simulink model "sampleModel1947"  (R2023a)
settings: Solver=VariableStepAuto  StartTime=0.0  StopTime=10.0  RelTol=1e-3
libraries: hdlsllib x7
settings Model: Creator=user1  LastModifiedBy=user1

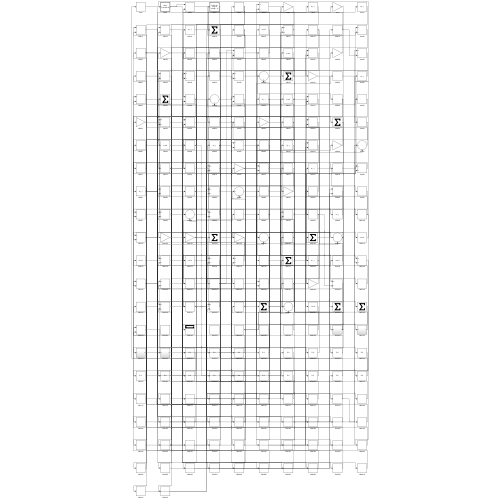
[thumbnail: Simulink's stored preview of the top-level diagram]
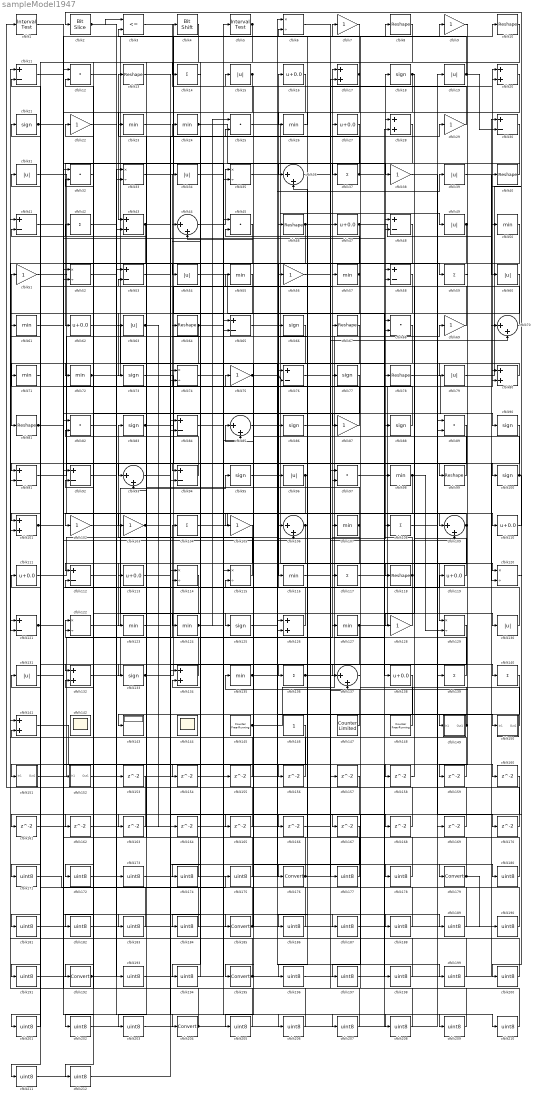
== system sampleModel1947 ==
  cfblk1 : hdlsllib/Logic and Bit Operations/Interval Test  IntervalClosedRight=on  uplimit=0.5  IntervalClosedLeft=on  lowlimit=-0.5  OutDataTypeStr=boolean
  cfblk{8,10,13,40,46,64,67,78,81,99,118} (11 alike) : Reshape
  cfblk{18,21,66,73,77,83,86,88,90,95,100,125,133} (13 alike) : Signum
  cfblk{17,20,28,43,80,101,126,132,134,141} (10 alike) : Sum
  cfblk{7,9,22,29,38,51,56,69,75,87,102..103,105,128} (14 alike) : Gain
  cfblk{14,37,42,59,104,108,117,136,139..140} (10 alike) : Sum  Inputs=+
  cfblk{36,44,70,85,93,106,109,137} (8 alike) : Sum  Inputs=|++
  cfblk{23..24,26,50,55,57,61,71..72,98,107,116,123..124,127,135} (16 alike) : MinMax
  cfblk{11,30,41,48,53,58,65,76,84,91..92,94,112,121} (14 alike) : Sum  Inputs=+-
  cfblk{16,27,47,62,110..111,113,119,138} (9 alike) : Bias  Bias=0.0  SaturateOnIntegerOverflow=off
  cfblk{6,33,35,52,74,114..115,120,122,129} (10 alike) : Product  Inputs=*/  RndMeth=Zero  SaturateOnIntegerOverflow=on
  cfblk{12,25,32,45,68,82,89,97} (8 alike) : DotProduct  OutDataTypeStr=Inherit: Inherit via internal rule
  cfblk{15,19,31,34,39,49,54,60,63,79,96,130..131} (13 alike) : Abs  SaturateOnIntegerOverflow=off
  cfblk142 : Scope
      settings: Floating=on
  cfblk143 : Display
  cfblk144 : Scope
      settings: Floating=on
  cfblk145 : hdlsllib/Sources/Counter Free-Running  NumBits=16  tsamp=-1
  cfblk146 : Constant  SampleTime=-1
  cfblk147 : hdlsllib/Sources/Counter Limited  uplimit=7  tsamp=-1
  cfblk148 : hdlsllib/Sources/Counter Free-Running  NumBits=16  tsamp=-1
  cfblk149 : Subsystem
      settings: LibrarySourceBlock=|
      | hdlsllib/Ports &
      | Subsystems/Subsystem
  cfblk150 : Subsystem
      settings: LibrarySourceBlock=|
      | hdlsllib/Ports &
      | Subsystems/Subsystem
  cfblk151 : Subsystem
      settings: LibrarySourceBlock=|
      | hdlsllib/Ports &
      | Subsystems/Subsystem
  cfblk152 : Subsystem
      settings: LibrarySourceBlock=|
      | hdlsllib/Ports &
      | Subsystems/Subsystem
  cfblk{153..170} (18 alike) : Delay  SampleTime=1
  cfblk{171..175,177..178,180..184,186..191,193..194,196..203,205..212} (36 alike) : DataTypeConversion  OutDataTypeStr=uint8  SaturateOnIntegerOverflow=off  RndMeth=Floor
  cfblk{176,179,185,192,195,204} (6 alike) : DataTypeConversion  SaturateOnIntegerOverflow=off  RndMeth=Floor
  cfblk2 : hdlsllib/Logic and Bit Operations/Bit Slice  lidx=7  ridx=0
  cfblk3 : RelationalOperator  Operator=<=  OutDataTypeStr=boolean  InputSameDT=off
  cfblk4 : hdlsllib/Logic and Bit Operations/Bit Shift  mode=Shift Left Logical  N=0
  cfblk5 : hdlsllib/Logic and Bit Operations/Interval Test  IntervalClosedRight=on  uplimit=0.5  IntervalClosedLeft=on  lowlimit=-0.5  OutDataTypeStr=boolean
  wires:
  cfblk136/1 -> cfblk69/1, cfblk137/2
  cfblk126/1 -> cfblk16/1
  cfblk151/1(Out1) -> cfblk17/1
  cfblk48/1 -> cfblk116/1
  cfblk106/1 -> cfblk136/1, cfblk156/1, cfblk194/1
  cfblk133/1 -> cfblk57/1, cfblk180/1
  cfblk40/1 -> cfblk37/1
  cfblk96/1 -> cfblk102/1, cfblk66/1
  cfblk25/1 -> cfblk129/1
  cfblk72/1 -> cfblk10/1, cfblk112/1, cfblk209/1
  cfblk79/1 -> cfblk2/1
  cfblk49/1 -> cfblk132/1, cfblk101/2
  cfblk118/1 -> cfblk18/1, cfblk112/2
  cfblk139/1 -> cfblk122/1
  cfblk31/1 -> cfblk94/1
  cfblk99/1 -> cfblk78/1
  cfblk132/1 -> cfblk127/1
  cfblk87/1 -> cfblk51/1
  cfblk51/1 -> cfblk139/1
  cfblk97/1 -> cfblk99/1
  cfblk27/1 -> cfblk62/1
  cfblk115/1 -> cfblk83/1
  cfblk43/1 -> cfblk151/1(In1), cfblk137/1
  cfblk78/1 -> cfblk135/1
  cfblk152/1(Out1) -> cfblk96/1
  cfblk127/1 -> cfblk20/1, cfblk212/1
  cfblk69/1 -> cfblk27/1
  cfblk94/1 -> cfblk42/1
  cfblk24/1 -> cfblk38/1, cfblk184/1
  cfblk104/1 -> cfblk106/1
  cfblk80/1 -> cfblk76/1
  cfblk3/1 -> cfblk65/2
  cfblk150/1(Out1) -> cfblk77/1
  cfblk102/1 -> cfblk130/1
  cfblk33/1 -> cfblk8/1
  cfblk71/1 -> cfblk21/1
  cfblk88/1 -> cfblk34/1
  cfblk134/1 -> cfblk104/1
  cfblk63/1 -> cfblk23/1, cfblk164/1
  cfblk59/1 -> cfblk149/1(In1)
  cfblk60/1 -> cfblk94/2
  cfblk35/1 -> cfblk49/1
  cfblk91/1 -> cfblk48/1
  cfblk103/1 -> cfblk109/1, cfblk188/1
  cfblk44/1 -> cfblk35/1
  cfblk61/1 -> cfblk185/1
  cfblk122/1 -> cfblk95/1
  cfblk58/1 -> cfblk73/1
  cfblk135/1 -> cfblk25/2, cfblk199/1
  cfblk149/1(Out1) -> cfblk56/1, cfblk117/1
  cfblk14/1 -> cfblk124/1
  cfblk2/1 -> cfblk3/1, cfblk35/2
  cfblk66/1 -> cfblk81/1
  cfblk117/1 -> cfblk19/1
  cfblk10/1 -> cfblk54/1
  cfblk123/1 -> cfblk125/1
  cfblk84/1 -> cfblk179/1
  cfblk70/1 -> cfblk31/1
  cfblk47/1 -> cfblk50/1, cfblk181/1
  cfblk119/1 -> cfblk58/1
  cfblk39/1 -> cfblk60/1
  cfblk62/1 -> cfblk126/2
  cfblk46/1 -> cfblk143/1, cfblk109/2
  cfblk81/1 -> cfblk80/1, cfblk106/2, cfblk87/1
  cfblk110/1 -> cfblk40/1
  cfblk1/1 -> cfblk59/1
  cfblk41/1 -> cfblk110/1
  cfblk75/1 -> cfblk76/2, cfblk67/1
  cfblk128/1 -> cfblk7/1
  cfblk108/1 -> cfblk80/2
  cfblk137/1 -> cfblk107/1
  cfblk54/1 -> cfblk98/1
  cfblk100/1 -> cfblk44/2, cfblk200/1
  cfblk20/1 -> cfblk26/1
  cfblk36/1 -> cfblk70/2
  cfblk56/1 -> cfblk47/1
  cfblk125/1 -> cfblk108/1
  cfblk29/1 -> cfblk4/1
  cfblk57/1 -> cfblk91/2, cfblk15/1, cfblk191/1
  cfblk18/1 -> cfblk128/1, cfblk63/1
  cfblk130/1 -> cfblk75/1
  cfblk68/1 -> cfblk195/1
  cfblk30/1 -> cfblk36/1
  cfblk65/1 -> cfblk138/1
  cfblk16/1 -> cfblk43/1
  cfblk19/1 -> cfblk3/2, cfblk30/2
  cfblk131/1 -> cfblk48/2
  cfblk109/1 -> cfblk105/1, cfblk163/1
  cfblk17/1 -> cfblk14/1, cfblk166/1
  cfblk26/1 -> cfblk6/2
  cfblk50/1 -> cfblk79/1
  cfblk21/1 -> cfblk152/1(In1), cfblk33/2
  cfblk5/1 -> cfblk93/2, cfblk174/1
  cfblk53/1 -> cfblk176/1
  cfblk76/1 -> cfblk120/1
  cfblk147/1 -> cfblk36/2
  cfblk90/1 -> cfblk120/2
  cfblk8/1 -> cfblk101/1
  cfblk37/1 -> cfblk29/1, cfblk13/1
  cfblk121/1 -> cfblk115/2, cfblk183/1
  cfblk124/1 -> cfblk119/1, cfblk140/1, cfblk25/1
  cfblk83/1 -> cfblk5/1, cfblk113/1
  cfblk55/1 -> cfblk71/1
  cfblk114/1 -> cfblk192/1
  cfblk113/1 -> cfblk28/1
  cfblk67/1 -> cfblk91/1
  cfblk28/1 -> cfblk103/1
  cfblk101/1 -> cfblk9/1, cfblk160/1
  cfblk107/1 -> cfblk123/1, cfblk41/2
  cfblk45/1 -> cfblk121/2
  cfblk6/1 -> cfblk118/1
  cfblk111/1 -> cfblk39/1
  cfblk92/1 -> cfblk204/1
  cfblk73/1 -> cfblk100/1
  cfblk64/1 -> cfblk93/1, cfblk90/1
  cfblk95/1 -> cfblk150/1(In1)
  cfblk7/1 -> cfblk133/1
  cfblk145/1 -> cfblk28/2, cfblk20/2
  cfblk15/1 -> cfblk72/1, cfblk52/2
  cfblk98/1 -> cfblk129/2, cfblk196/1
  cfblk148/1 -> cfblk55/1
  cfblk82/1 -> cfblk153/1
  cfblk153/1 -> cfblk1/1
  cfblk42/1 -> cfblk154/1
  cfblk154/1 -> cfblk45/1
  cfblk34/1 -> cfblk155/1
  cfblk155/1 -> cfblk121/1
  cfblk156/1 -> cfblk65/1
  cfblk116/1 -> cfblk158/1
  cfblk158/1 -> cfblk58/2
  cfblk9/1 -> cfblk159/1
  cfblk159/1 -> cfblk126/1
  cfblk129/1 -> cfblk161/1
  cfblk161/1 -> cfblk17/2
  cfblk105/1 -> cfblk162/1
  cfblk162/1 -> cfblk43/2
  cfblk163/1 -> cfblk132/2
  cfblk164/1 -> cfblk6/1
  cfblk23/1 -> cfblk165/1
  cfblk165/1 -> cfblk44/1
  cfblk120/1 -> cfblk167/1
  cfblk13/1 -> cfblk168/1
  cfblk168/1 -> cfblk41/1
  cfblk169/1 -> cfblk115/1
  cfblk38/1 -> cfblk170/1
  cfblk170/1 -> cfblk24/1
  cfblk157/1 -> cfblk171/1
  cfblk77/1 -> cfblk172/1
  cfblk172/1 -> cfblk157/1
  cfblk12/1 -> cfblk173/1
  cfblk173/1 -> cfblk86/1
  cfblk174/1 -> cfblk12/1
  cfblk171/1 -> cfblk175/1
  cfblk175/1 -> cfblk12/2
  cfblk176/1 -> cfblk134/2, cfblk64/1
  cfblk86/1 -> cfblk177/1
  cfblk177/1 -> cfblk53/1
  cfblk166/1 -> cfblk178/1
  cfblk178/1 -> cfblk53/2
  cfblk179/1 -> cfblk46/1, cfblk190/1
  cfblk180/1 -> cfblk84/1
  cfblk181/1 -> cfblk84/2
  cfblk32/1 -> cfblk182/1
  cfblk182/1 -> cfblk70/1
  cfblk183/1 -> cfblk32/1
  cfblk184/1 -> cfblk32/2
  cfblk185/1 -> cfblk45/2, cfblk82/1
  cfblk138/1 -> cfblk186/1
  cfblk186/1 -> cfblk61/1
  cfblk22/1 -> cfblk187/1
  cfblk187/1 -> cfblk169/1
  cfblk188/1 -> cfblk22/1
  cfblk85/1 -> cfblk189/1
  cfblk189/1 -> cfblk111/1
  cfblk190/1 -> cfblk85/1
  cfblk191/1 -> cfblk85/2
  cfblk192/1 -> cfblk33/1, cfblk82/2
  cfblk52/1 -> cfblk193/1
  cfblk193/1 -> cfblk114/1
  cfblk194/1 -> cfblk114/2
  cfblk195/1 -> cfblk52/1, cfblk30/1
  cfblk196/1 -> cfblk68/1
  cfblk160/1 -> cfblk197/1
  cfblk197/1 -> cfblk68/2
  cfblk141/1 -> cfblk198/1
  cfblk198/1 -> cfblk122/2
  cfblk199/1 -> cfblk141/1
  cfblk200/1 -> cfblk141/2
  cfblk89/1 -> cfblk201/1
  cfblk201/1 -> cfblk131/1
  cfblk4/1 -> cfblk202/1
  cfblk202/1 -> cfblk89/1
  cfblk140/1 -> cfblk203/1
  cfblk203/1 -> cfblk89/2
  cfblk204/1 -> cfblk134/1, cfblk88/1
  cfblk167/1 -> cfblk205/1
  cfblk205/1 -> cfblk92/1
  cfblk93/1 -> cfblk206/1
  cfblk206/1 -> cfblk92/2
  cfblk11/1 -> cfblk207/1
  cfblk207/1 -> cfblk97/1
  cfblk112/1 -> cfblk208/1
  cfblk208/1 -> cfblk11/1
  cfblk209/1 -> cfblk11/2
  cfblk74/1 -> cfblk210/1
  cfblk210/1 -> cfblk97/2
  cfblk146/1 -> cfblk211/1
  cfblk211/1 -> cfblk74/1
  cfblk212/1 -> cfblk74/2

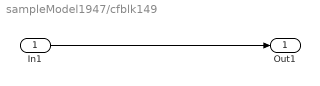
== system sampleModel1947/cfblk149 ==
  In1 : Inport
  Out1 : Outport
  wires:
  In1/1 -> Out1/1

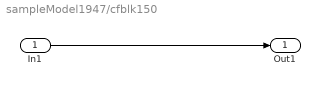
== system sampleModel1947/cfblk150 ==
  In1 : Inport
  Out1 : Outport
  wires:
  In1/1 -> Out1/1

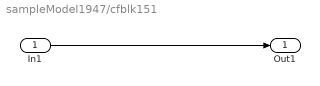
== system sampleModel1947/cfblk151 ==
  In1 : Inport
  Out1 : Outport
  wires:
  In1/1 -> Out1/1

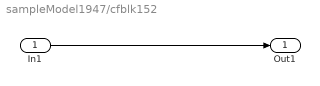
== system sampleModel1947/cfblk152 ==
  In1 : Inport
  Out1 : Outport
  wires:
  In1/1 -> Out1/1
